simulink model "PruebaDeadZone"  (R2021b)
settings: Solver=FixedStepAuto  StartTime=0.0  StopTime=20  RelTol=1e-3  EnableMultiTasking=on
libraries: SignalEditorBlockLib x1
settings Model: ExtModeTrigDuration=2  Creator=yo  LastModifiedBy=yo
settings OptimizationCC: EnhancedBackFolding=on  PassReuseOutputArgsAs=Individual arguments  ZeroExternalMemoryAtStartup=off  ZeroInternalMemoryAtStartup=off  MaxStackSize=64  OptimizeBlockOrder=speed  DifferentSizesBufferReuse=on  OptimizationCustomize=off  EfficientTunableParamExpr=on
settings DebuggingCC: ParameterTunabilityLossMsg=error
settings HardwareCC: ProdBitPerInt=16  ProdBitPerPointer=16  ProdBitPerSizeT=16  ProdBitPerPtrDiffT=16  ProdLargestAtomicFloat=None  ProdWordSize=8  ProdHWDeviceType=Atmel->AVR  UseEmbeddedCoderFeatures=off  UseSimulinkCoderFeatures=off
settings SFSimCC: MATLABDynamicMemAlloc=off
settings RTWCC: Description=Embedded Coder  SystemTargetFile=ert.tlc  HardwareBoard=Arduino Mega 2560  TemplateMakefile=ert_default_tmf  Toolchain=Arduino AVR  BuildConfiguration=Faster Runs
settings CodeAppCC: ForceParamTrailComments=on  IgnoreCustomStorageClasses=off  OperatorAnnotations=on  SimulinkDataObjDesc=on  SFDataObjDesc=on  MangleLength=10  InsertBlockDesc=on
settings ERTTargetCC: SupportContinuousTime=on  SupportNonInlinedSFcns=on  SupportVariableSizeSignals=on  ExtModeTransport=3  ExtModeStaticAlloc=on  ExtModeStaticAllocSize=2048  ExtModeMexFile=ext_xcp  ExtModeIntrfLevel=Level2 - Open

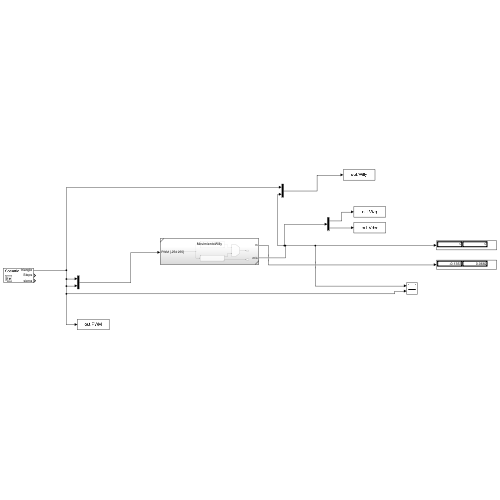
[thumbnail: Simulink's stored preview of the top-level diagram]
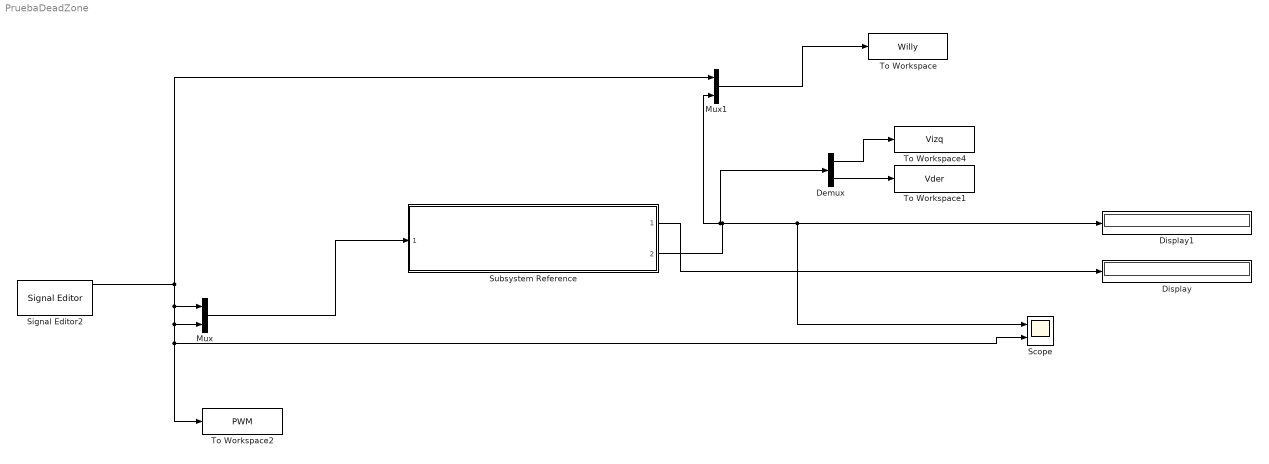
== system PruebaDeadZone ==
  Demux : Demux  Outputs=2
  Display : Display
  Display1 : Display
  Mux : Mux  Inputs=2
  Mux1 : Mux  Inputs=2
  Scope : Scope  NumInputPorts=2
  Signal Editor2 : SignalEditorBlockLib/Signal Editor  FileName=C:\Users\yo\Git\Willy_LabRob\ProjectoWilly\Senales de prueba\Signals.mat  ActiveScenario=Scenario  ActiveSignal=triangle  IsBus=off  OutputBusObjectStr=Bus: BusObject  SampleTime=0.01  ZeroCross=off  OutputAfterFinalValue=Setting to zero  Unit=inherit  PreserveSignalName=on
  Subsystem Reference : Subsystem  ReferencedSubsystem=MovimientoWilly
  To Workspace : ToWorkspace  VariableName=Willy  SampleTime=-1
      settings: Save2DSignal=2-D array (concatenate along first dimension)
  To Workspace1 : ToWorkspace  VariableName=Vder  SampleTime=-1
      settings: Save2DSignal=2-D array (concatenate along first dimension)
  To Workspace2 : ToWorkspace  VariableName=PWM  SampleTime=-1
      settings: Save2DSignal=2-D array (concatenate along first dimension)
  To Workspace4 : ToWorkspace  VariableName=Vizq  SampleTime=-1
      settings: Save2DSignal=2-D array (concatenate along first dimension)
  wires:
  Subsystem Reference/2 -> Demux/1, Mux1/2, Scope/1, Display1/1
  Mux/1 -> Subsystem Reference/1
  Signal Editor2/1 -> Scope/2, To Workspace2/1, Mux/2, Mux/1, Mux1/1
  Mux1/1 -> To Workspace/1
  Subsystem Reference/1 -> Display/1
  Demux/1 -> To Workspace4/1
  Demux/2 -> To Workspace1/1
